simulink model "ACC_T_staliro"  (R2024b)
settings: Solver=FixedStepAuto  StartTime=0.0  StopTime=T  RelTol=1e-3
undefined symbols (not defined in the file): D_default, t_gap, Ts, v0_ego, v0_lead, v_set, x0_ego, x0_lead
libraries: mpcadaslib x1
settings Model: Creator=The MathWorks, Inc.  LastModifiedBy=quandoan
settings SolverCC: AlgebraicLoopSolver=TrustRegion
settings DataIOCC: ExternalInput=inputTimeseries  LoadExternalInput=on  SaveFormat=Array  ReturnWorkspaceOutputs=off
settings DebuggingCC: UnconnectedInputMsg=warning  UnconnectedOutputMsg=warning  UnconnectedLineMsg=warning  ArithmeticOperatorsInVariantConditions=warning
settings ModelReferenceCC: EnableRefExpFcnMdlSchedulingChecks=on
settings SFSimCC: SimUseLocalCustomCode=off  CustomCodeUndefinedFunction=UseInterfaceOnly
settings RTWCC: RTWUseLocalCustomCode=off  GPUComputeCapability=3.5  DLArmComputeVersion=19.05
settings CodeAppCC: StateflowObjectComments=on

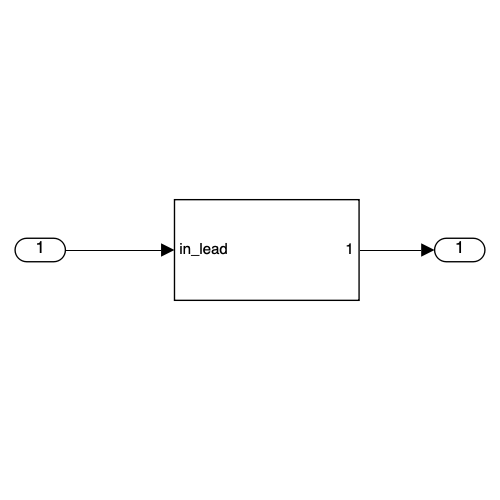
[thumbnail: Simulink's stored preview of the top-level diagram]
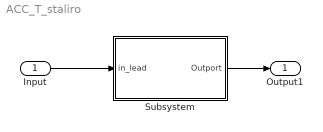
== system ACC_T_staliro ==
  Input : Inport
  Subsystem : Subsystem
  Output1 : Outport
  wires:
  Input/1 -> Subsystem/1(in_lead)
  Subsystem/1(Outport) -> Output1/1

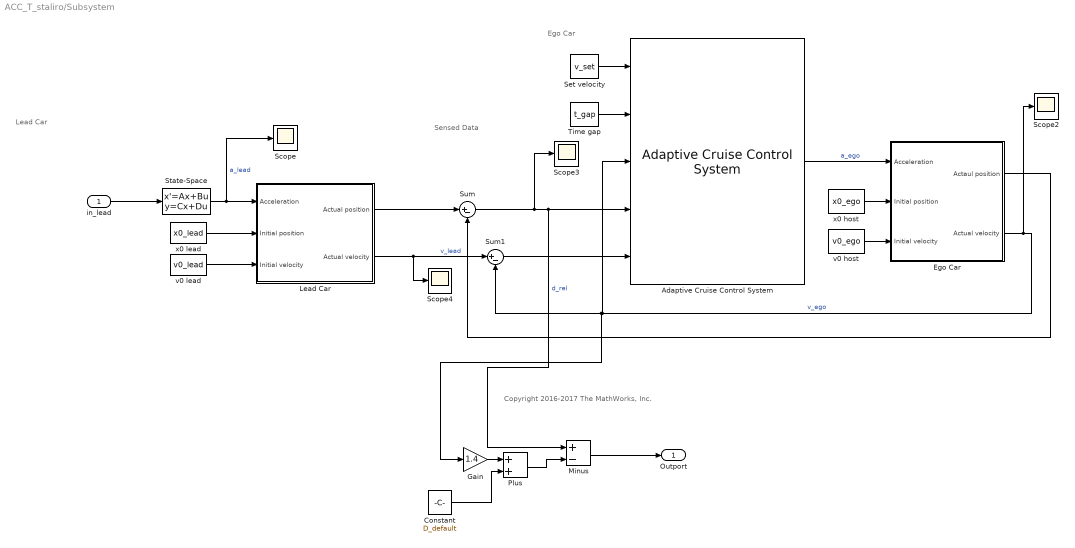
== system ACC_T_staliro/Subsystem ==
  note: Sensed Data
  note: Lead Car
  note: Ego Car
  note: Copyright 2016-2017 The MathWorks, Inc.
  in_lead : Inport
  Adaptive Cruise Control System : mpcadaslib/Adaptive Cruise Control System  EgoModel=tf(1,[0.5,1,0])  InitialEgoVelocity=v0_ego  DefaultSpacing=D_default  MaxVelocity=50  MinAcceleration=-3  amin_ext=off  MaxAcceleration=2  amax_ext=off  Ts=0.1  PredictionHorizon=30  ControllerBehavior=0.0  suboptimal=off  maxiter=10  datatypeopt=double  optmode=off  trackmode=off
  Constant : Constant  Value=D_default
  Ego Car : Subsystem
  Gain : Gain  Gain=1.4
  Lead Car : Subsystem
  Minus : Sum  Inputs=+-
  Plus : Sum
  Scope{,2..4} (4 alike) : Scope
  Set velocity : Constant  Value=v_set  SampleTime=Ts
  State-Space : StateSpace  A=-10  B=10  D=0  InitialCondition=0
  Sum : Sum  Inputs=|+-
  Sum1 : Sum  Inputs=|+-
  Time gap : Constant  Value=t_gap  SampleTime=Ts
  v0 host : Constant  Value=v0_ego  SampleTime=Ts
  v0 lead : Constant  Value=v0_lead  SampleTime=Ts
  x0 host : Constant  Value=x0_ego  SampleTime=Ts
  x0 lead : Constant  Value=x0_lead  SampleTime=Ts
  Outport : Outport
  wires:
  Gain/1 -> Plus/1
  Sum1/1 -> Adaptive Cruise Control System/5
  Minus/1 -> Outport/1
  Ego Car/1(Actaul position) -> Sum/2
  in_lead/1 -> State-Space/1
  Ego Car/2(Actual velocity) -> Scope2/1, Adaptive Cruise Control System/3, Gain/1, Sum1/2  "v_ego"
  Sum/1 -> Scope3/1, Minus/1, Adaptive Cruise Control System/4  "d_rel"
  Adaptive Cruise Control System/1 -> Ego Car/1(Acceleration)  "a_ego"
  Constant/1 -> Plus/2
  Time gap/1 -> Adaptive Cruise Control System/2
  Plus/1 -> Minus/2
  Lead Car/1(Actual position) -> Sum/1
  State-Space/1 -> Scope/1, Lead Car/1(Acceleration)  "a_lead"
  v0 lead/1 -> Lead Car/3(Initial velocity)
  x0 host/1 -> Ego Car/2(Initial position)
  x0 lead/1 -> Lead Car/2(Initial position)
  v0 host/1 -> Ego Car/3(Initial velocity)
  Lead Car/2(Actual velocity) -> Scope4/1, Sum1/1  "v_lead"
  Set velocity/1 -> Adaptive Cruise Control System/1

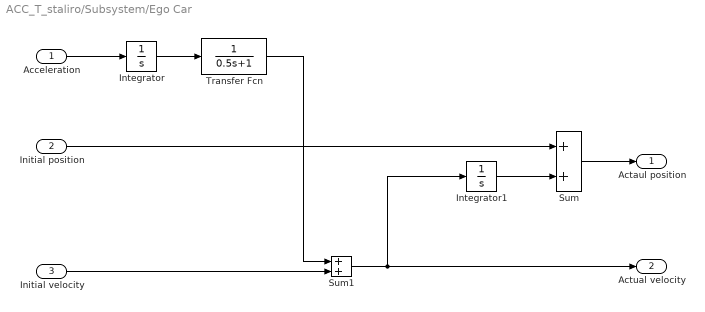
== system ACC_T_staliro/Subsystem/Ego Car ==
  Acceleration : Inport
  Initial position : Inport  Port=2
  Initial velocity : Inport  Port=3
  Integrator : Integrator
  Integrator1 : Integrator
  Sum : Sum
  Sum1 : Sum
  Transfer Fcn : TransferFcn  Denominator=[0.5 1]
  Actaul position : Outport  VectorParamsAs1DForOutWhenUnconnected=off
  Actual velocity : Outport  Port=2  VectorParamsAs1DForOutWhenUnconnected=off
  wires:
  Sum1/1 -> Integrator1/1, Actual velocity/1
  Initial velocity/1 -> Sum1/2
  Sum/1 -> Actaul position/1
  Transfer Fcn/1 -> Sum1/1
  Integrator/1 -> Transfer Fcn/1
  Acceleration/1 -> Integrator/1
  Initial position/1 -> Sum/1
  Integrator1/1 -> Sum/2

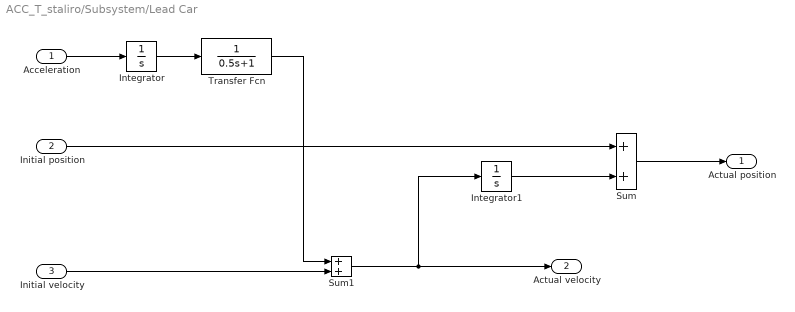
== system ACC_T_staliro/Subsystem/Lead Car ==
  Acceleration : Inport
  Initial position : Inport  Port=2
  Initial velocity : Inport  Port=3
  Integrator : Integrator
  Integrator1 : Integrator
  Sum : Sum
  Sum1 : Sum
  Transfer Fcn : TransferFcn  Denominator=[0.5 1]
  Actual position : Outport  VectorParamsAs1DForOutWhenUnconnected=off
  Actual velocity : Outport  Port=2  VectorParamsAs1DForOutWhenUnconnected=off
  wires:
  Transfer Fcn/1 -> Sum1/1
  Initial velocity/1 -> Sum1/2
  Sum/1 -> Actual position/1
  Integrator/1 -> Transfer Fcn/1
  Sum1/1 -> Integrator1/1, Actual velocity/1
  Acceleration/1 -> Integrator/1
  Initial position/1 -> Sum/1
  Integrator1/1 -> Sum/2
